simulink model "q_heli3d_semestral_project_FL"  (Simulink 8.9)
settings: Solver=ode1  StartTime=0.0  StopTime=inf  FixedStep=0.002  RelTol=1e-3  EnableMultiTasking=on
values from neighbouring files (symbols this model uses):
  ae1 = model_identified.Parameters(3).Value    [model_benchmark_init.m]    (also in workspace.mat = 1.36231449822)
  ae2 = model_identified.Parameters(4).Value    [model_benchmark_init.m]    (also in workspace.mat = -0.378717172069)
  at = model_identified.Parameters(7).Value    [model_benchmark_init.m]    (also in workspace.mat = -0.463804529993)
  be = model_identified.Parameters(6).Value    [model_benchmark_init.m]    (also in workspace.mat = 0.116311837295)
  bl = model_identified.Parameters(2).Value    [model_benchmark_init.m]    (also in workspace.mat = 0.103160863637)
  bt = model_identified.Parameters(9).Value    [model_benchmark_init.m]    (also in workspace.mat = 0.962119048974)
  ce = model_identified.Parameters(5).Value    [model_benchmark_init.m]    (also in workspace.mat = 0.04469700002)
  cl = model_identified.Parameters(1).Value    [model_benchmark_init.m]    (also in workspace.mat = 0.202457747385)
  ct = model_identified.Parameters(8).Value    [model_benchmark_init.m]    (also in workspace.mat = 0.00762763482449)
  elev_0 = -0.479965544298    [workspace.mat]
  K_AMP = 3    [workspace.mat]
  K_EC_E = -0.00153398078789    [workspace.mat]
  K_EC_P = 0.00153398078789    [workspace.mat]
  K_EC_T = 0.000766990393943    [workspace.mat]
  par_ctrl =     [workspace.mat]
  par_id = struct    [model_benchmark_init.m]    (also in workspace.mat = )
  VMAX_AMP = 24    [workspace.mat]
  VMAX_DAC = 10    [workspace.mat]
  wcf = 125.663706144    [workspace.mat]
  x0 = [0; 0; 0; 0; 0; 0]    [model_benchmark_init.m]    (also in model_benchmark_ode45.m = [0; 0; 0; 0; 0.1; 0]; workspace.mat = [0 0 0.1745 0 -0.1047 0])
  zetaf = 0.9    [workspace.mat]
undefined symbols (not defined in the file or in its folder): HIL, qc_get_step_size
libraries: quarc_library x4, simulink_extras x4
settings Model: Creator=MLevis  LastModifiedBy=obrusvit  SimulationMode=external  ExtModeTrigDuration=1000000
settings SolverCC: PositivePriorityOrder=on
settings DataIOCC: MaxDataPoints=100000
settings OptimizationCC: ExpressionDepthLimit=2147483647  InitFltsAndDblsToZero=on
settings DebuggingCC: SaveWithParameterizedLinksMsg=none  SolverPrmCheckMsg=warning
settings RTWCC: SystemTargetFile=quarc_win64.tlc  TemplateMakefile=quarc_default_tmf  Description=QUARC Win64 Target
settings STFCustomTargetCC: TargetPreCompLibLocation=C:\PROGRA~3\QUARC\lib\2017a\win64\release  ConcurrentExecutionCompliant=on  GeneratePreprocessorConditionals=Disable all  SystemTargetFile=quarc_win64.tlc
settings GRTTargetCC: TargetPreCompLibLocation=C:\PROGRA~3\QUARC\lib\2017a\win64\release  ParMdlRefBuildCompliant=off  CompOptLevelCompliant=off  MatFileLogging=off  CPPClassGenCompliant=off  UseToolchainInfoCompliant=off  ExtMode=on  ExtModeMexFile=quarc_comm

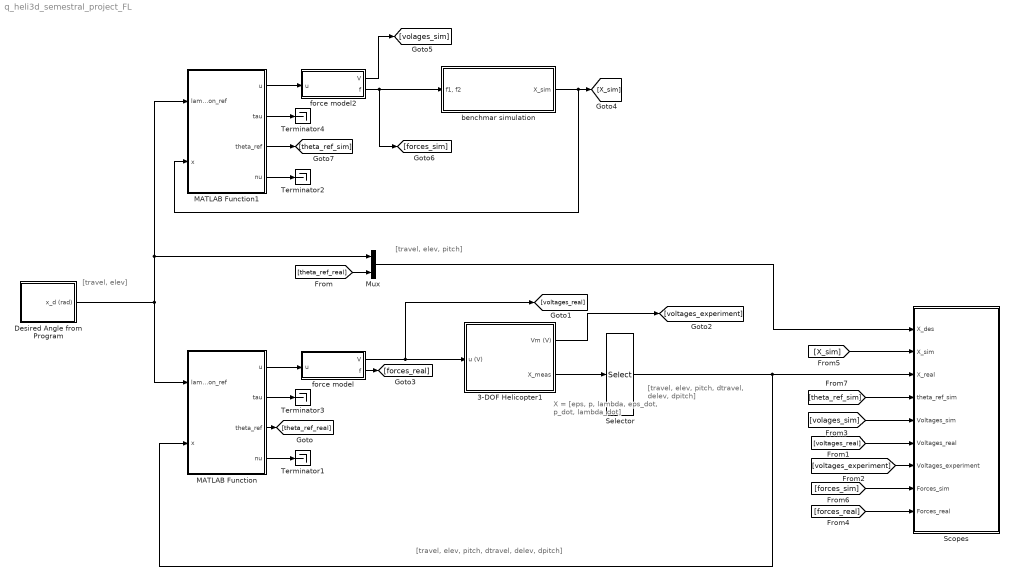
== system q_heli3d_semestral_project_FL ==
  note: [travel, elev]
  note: [travel, elev, pitch, dtravel, delev, dpitch]
  note: [travel, elev, pitch]
  note: X = [eps, p, lambda, eps_dot, p_dot, lambda_dot]
  note: [travel, elev, pitch, dtravel, delev, dpitch]
  3-DOF Helicopter1 : Subsystem
  Desired Angle from Program : Subsystem
  MATLAB Function : MATLAB Function  TreatAsAtomicUnit=on
  MATLAB Function1 : MATLAB Function  TreatAsAtomicUnit=on
  Mux : Mux  Inputs=2
  Scopes : Subsystem
  Selector : Selector  InputPortWidth=6  IndexOptions=Index vector (dialog)  Indices=[3 1 2 6 4 5]  OutputSizes=1
  Terminator{1..4} (4 alike) : Terminator
  benchmar simulation : Subsystem
  force model : Subsystem
  force model2 : Subsystem
  wires:
  Mux/1 -> Scopes/1(X_des)
  [theta_ref_real] -> Mux/2
  MATLAB Function/2(tau) -> Terminator3/1
  MATLAB Function/4(nu) -> Terminator1/1
  force model/2(f) -> [forces_real]
  MATLAB Function/3(theta_ref) -> [theta_ref_real]
  Desired Angle from Program/1(x_d (rad)) -> MATLAB Function/1(lambda_epsilon_ref), Mux/1, MATLAB Function1/1(lambda_epsilon_ref)
  [forces_real] -> Scopes/9("Forces_real ")
  [voltages_real] -> Scopes/6("Voltages_real ")
  MATLAB Function/1(u) -> force model/1(u)
  3-DOF Helicopter1/2(X_meas) -> Selector/1
  Selector/1 -> MATLAB Function/2(x), Scopes/3("X_real ")
  [X_sim] -> Scopes/2(X_sim)
  force model2/2(f) -> benchmar simulation/1("f1, f2"), [forces_sim]
  benchmar simulation/1("X_sim ") -> MATLAB Function1/2(x), [X_sim]
  force model/1(V) -> [voltages_real], 3-DOF Helicopter1/1(u (V))
  MATLAB Function1/1(u) -> force model2/1(u)
  MATLAB Function1/4(nu) -> Terminator2/1
  MATLAB Function1/3(theta_ref) -> [theta_ref_sim]
  MATLAB Function1/2(tau) -> Terminator4/1
  force model2/1(V) -> [volages_sim]
  [volages_sim] -> Scopes/5(Voltages_sim)
  [forces_sim] -> Scopes/8(Forces_sim)
  [theta_ref_sim] -> Scopes/4("theta_ref_sim ")
  3-DOF Helicopter1/1(Vm (V)) -> [voltages_experiment]
  [voltages_experiment] -> Scopes/7(Voltages_experiment)

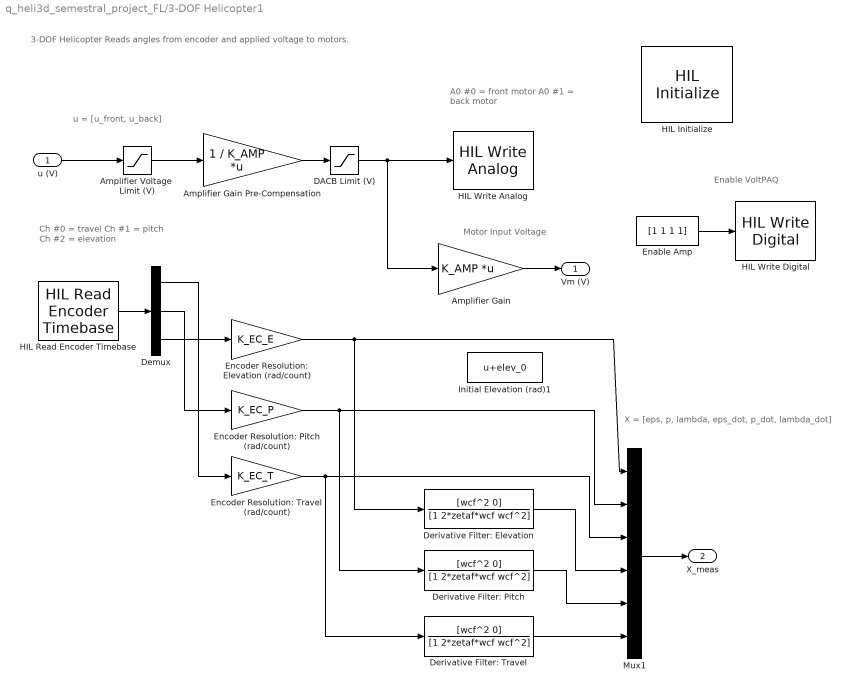
== system q_heli3d_semestral_project_FL/3-DOF Helicopter1 ==
  note: Enable VoltPAQ
  note: X = [eps, p, lambda, eps_dot, p_dot, lambda_dot]
  note: Ch #0 = travel
      | Ch #1 = pitch
      | Ch #2 = elevation
  note: 3-DOF Helicopter
      | Reads angles from encoder and applied voltage to motors.
  note: Motor Input Voltage
  note: u = [u_front, u_back]
  note: A0 #0 = front motor
      | A0 #1 = back motor
  u (V) : Inport
  Amplifier Gain : Gain  Gain=K_AMP  Multiplication=Matrix(K*u)  SaturateOnIntegerOverflow=on  OutDataTypeStr=Inherit: Same as input  ParamDataTypeStr=Inherit: Same as input
  Amplifier Gain Pre-Compensation : Gain  Gain=1 / K_AMP  Multiplication=Matrix(K*u)  SaturateOnIntegerOverflow=on  OutDataTypeStr=Inherit: Same as input  ParamDataTypeStr=Inherit: Same as input
  Amplifier Voltage  Limit (V) : Saturate  UpperLimit=VMAX_AMP  LowerLimit=-VMAX_AMP
  DACB Limit (V) : Saturate  UpperLimit=VMAX_DAC  LowerLimit=-VMAX_DAC
  Demux : Demux  Outputs=3
  Derivative Filter: Elevation : TransferFcn  Numerator=[wcf^2 0]  Denominator=[1 2*zetaf*wcf wcf^2]
  Derivative Filter: Pitch : TransferFcn  Numerator=[wcf^2 0]  Denominator=[1 2*zetaf*wcf wcf^2]
  Derivative Filter: Travel : TransferFcn  Numerator=[wcf^2 0]  Denominator=[1 2*zetaf*wcf wcf^2]
  Enable Amp : Constant  Value=[1 1 1 1]
  Encoder Resolution: Elevation (rad/count) : Gain  Gain=K_EC_E
  Encoder Resolution: Pitch (rad/count) : Gain  Gain=K_EC_P
  Encoder Resolution: Travel (rad/count) : Gain  Gain=K_EC_T
  HIL Initialize : quarc_library/Data Acquisition/Generic/Configuration/HIL Initialize  object_name=HIL-1  board_type=q8_usb  board_number=0  board_options=update_rate=normal;decimation=1  exclusive=off  active=on  hardware_clocks=[0:2]  clock_modes=[]  initial_clock_frequencies=[]  set_clock_params_at_start=off  set_clock_params_at_switch_in=off  set_clock_frequencies_at_start=off  set_clock_frequencies_at_switch_in=off  analog_input_channels=[0:7]  analog_input_configurations=[]  analog_input_maximums=10  analog_input_minimums=-10  set_analog_input_params_at_start=on  set_analog_input_params_at_switch_in=off  analog_output_channels=[0:7]  analog_output_maximums=10  analog_output_minimums=-10  initial_analog_outputs=[0]  final_analog_outputs=[0]  watchdog_analog_outputs=0  set_analog_output_params_at_start=on  set_analog_output_params_at_switch_in=off  set_analog_outputs_at_start=on  set_analog_outputs_at_switch_in=off  set_analog_outputs_at_terminate=on  set_analog_outputs_at_switch_out=off  set_analog_outputs_on_watchdog=off  digital_input_channels=[]  digital_output_channels=[]  digital_output_configuration=[]  initial_digital_outputs=[1]  final_digital_outputs=[1]  watchdog_digital_outputs=[1]  set_digital_output_params_at_start=off  set_digital_output_params_at_switch_in=off  set_digital_outputs_at_start=on  set_digital_outputs_at_switch_in=off  set_digital_outputs_at_terminate=on  set_digital_outputs_at_switch_out=off  set_digital_outputs_on_watchdog=off  encoder_channels=[0:7]  quadrature=[4]  encoder_filter_frequency=[]  initial_encoder_counts=[0]  set_encoder_params_at_start=on  set_encoder_params_at_switch_in=off  set_encoder_counts_at_start=on  set_encoder_counts_at_switch_in=off  pwm_channels=[0:7]  pwm_modes=0  pwm_frequency=99.532799999999995e6/4095  pwm_configuration=[0]  pwm_alignment=[0]  pwm_polarity=[1]  pwm_leading_deadband=[0]  pwm_trailing_deadband=[0]  initial_pwm_outputs=[0]  final_pwm_outputs=[0]  watchdog_pwm_outputs=[0]  set_pwm_params_at_start=on  set_pwm_params_at_switch_in=off  set_pwm_outputs_at_start=on  set_pwm_outputs_at_switch_in=off  set_pwm_outputs_at_terminate=on  set_pwm_outputs_at_switch_out=off  set_pwm_outputs_on_watchdog=off  other_output_channels=[]  initial_other_outputs=[]  final_other_outputs=[]  watchdog_other_outputs=[]  set_other_outputs_at_start=off  set_other_outputs_at_switch_in=off  set_other_outputs_at_terminate=off  set_other_outputs_at_switch_out=off  set_other_outputs_on_watchdog=off
  HIL Read Encoder Timebase : quarc_library/Data Acquisition/Generic/Timebases/HIL Read Encoder Timebase  object_name=HIL-1  clock=0  channels=[0:2]  samples_in_buffer=max(ceil(1/qc_get_step_size), 1)  active=on  vector_output=on  data_type_mode=Inherit via back propagation  data_type=double
  HIL Write Analog : quarc_library/Data Acquisition/Generic/Immediate I//O/HIL Write Analog  object_name=HIL-1  channels=[0,1]  sample_time=-1  active=off  vector_input=on
  HIL Write Digital : quarc_library/Data Acquisition/Generic/Immediate I//O/HIL Write Digital  object_name=HIL-1  channels=[0:3]  sample_time=-1  active=off  vector_input=on
      settings: SourceProductName=QUARC Targets
  Initial Elevation (rad)1 : Bias  Bias=elev_0
  Mux1 : Mux  Inputs=6
  Vm (V) : Outport
  X_meas : Outport  Port=2
  wires:
  Enable Amp/1 -> HIL Write Digital/1
  Encoder Resolution: Elevation (rad/count)/1 -> Mux1/1, Derivative Filter: Elevation/1
  Derivative Filter: Travel/1 -> Mux1/6
  Derivative Filter: Pitch/1 -> Mux1/5
  Derivative Filter: Elevation/1 -> Mux1/4
  Encoder Resolution: Travel (rad/count)/1 -> Derivative Filter: Travel/1, Mux1/3
  Encoder Resolution: Pitch (rad/count)/1 -> Derivative Filter: Pitch/1, Mux1/2
  Demux/2 -> Encoder Resolution: Pitch (rad/count)/1
  Demux/1 -> Encoder Resolution: Travel (rad/count)/1
  Demux/3 -> Encoder Resolution: Elevation (rad/count)/1
  DACB Limit (V)/1 -> HIL Write Analog/1, Amplifier Gain/1
  u (V)/1 -> Amplifier Voltage  Limit (V)/1
  Amplifier Gain/1 -> Vm (V)/1
  Amplifier Voltage  Limit (V)/1 -> Amplifier Gain Pre-Compensation/1
  Amplifier Gain Pre-Compensation/1 -> DACB Limit (V)/1
  Mux1/1 -> X_meas/1
  HIL Read Encoder Timebase/1 -> Demux/1

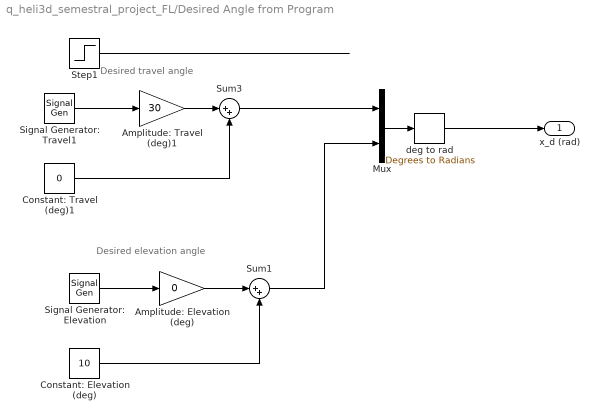
== system q_heli3d_semestral_project_FL/Desired Angle from Program ==
  note: Desired elevation angle
  note: Desired travel angle
  Amplitude: Elevation (deg) : Gain  Gain=0
  Amplitude: Travel (deg)1 : Gain  Gain=30
  Constant: Elevation (deg) : Constant  Value=10
  Constant: Travel (deg)1 : Constant  Value=0
  Mux : Mux  Inputs=2
  Signal Generator: Elevation : SignalGenerator  WaveForm=square  Frequency=0.04
  Signal Generator: Travel1 : SignalGenerator  WaveForm=square  Frequency=0.02
  Step1 : Step  Time=20  After=180  SampleTime=0
  Sum1 : Sum  Inputs=|++
  Sum3 : Sum  Inputs=|++
  deg to rad : simulink_extras/Transformations/Degrees to Radians
  x_d (rad) : Outport
  wires:
  Mux/1 -> deg to rad/1
  Constant: Elevation (deg)/1 -> Sum1/2
  Amplitude: Elevation (deg)/1 -> Sum1/1
  Signal Generator: Elevation/1 -> Amplitude: Elevation (deg)/1
  Sum1/1 -> Mux/2
  deg to rad/1 -> x_d (rad)/1
  Sum3/1 -> Mux/1
  Signal Generator: Travel1/1 -> Amplitude: Travel (deg)1/1
  Constant: Travel (deg)1/1 -> Sum3/2
  Amplitude: Travel (deg)1/1 -> Sum3/1
  Step1/1 -> ?

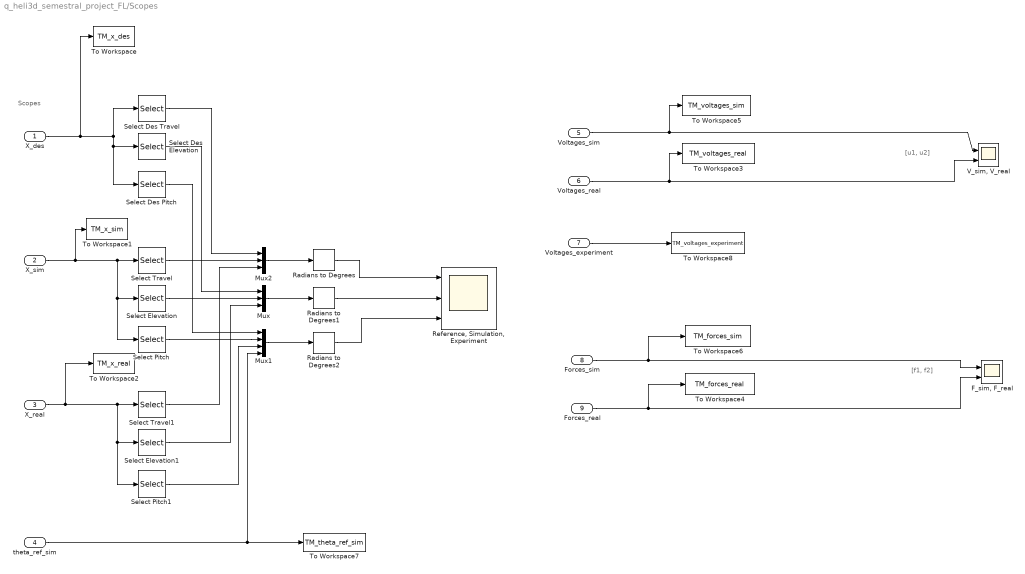
== system q_heli3d_semestral_project_FL/Scopes ==
  note: Scopes
  note: [f1, f2]
  note: [u1, u2]
  X_des : Inport
  X_sim : Inport  Port=2
  "X_real " : Inport  Port=3
  "theta_ref_sim " : Inport  Port=4
  Voltages_sim : Inport  Port=5
  "Voltages_real " : Inport  Port=6
  Voltages_experiment : Inport  Port=7
  Forces_sim : Inport  Port=8
  "Forces_real " : Inport  Port=9
  "F_sim, F_real" : Scope  NumInputPorts=2
  Mux : Mux  Inputs=3
  Mux1 : Mux
  Mux2 : Mux  Inputs=3
  Radians to Degrees : simulink_extras/Transformations/Radians to Degrees
  Radians to Degrees1 : simulink_extras/Transformations/Radians to Degrees
  Radians to Degrees2 : simulink_extras/Transformations/Radians to Degrees
  "Reference, Simulation, Experiment" : Scope  NumInputPorts=3
  Select Des Elevation : Selector  InputPortWidth=3  IndexOptions=Index vector (dialog)  Indices=2  OutputSizes=1
  Select Des Pitch : Selector  InputPortWidth=3  IndexOptions=Index vector (dialog)  Indices=3  OutputSizes=1
  Select Des Travel : Selector  InputPortWidth=3  IndexOptions=Index vector (dialog)  Indices=1  OutputSizes=1
  Select Elevation : Selector  InputPortWidth=6  IndexOptions=Index vector (dialog)  Indices=2  OutputSizes=1
  Select Elevation1 : Selector  InputPortWidth=6  IndexOptions=Index vector (dialog)  Indices=2  OutputSizes=1
  Select Pitch : Selector  InputPortWidth=6  IndexOptions=Index vector (dialog)  Indices=3  OutputSizes=1
  Select Pitch1 : Selector  InputPortWidth=6  IndexOptions=Index vector (dialog)  Indices=3  OutputSizes=1
  Select Travel : Selector  InputPortWidth=6  IndexOptions=Index vector (dialog)  Indices=1  OutputSizes=1
  Select Travel1 : Selector  InputPortWidth=6  IndexOptions=Index vector (dialog)  Indices=1  OutputSizes=1
  To Workspace : ToWorkspace  VariableName=TM_x_des  SampleTime=-1
  To Workspace1 : ToWorkspace  VariableName=TM_x_sim  SampleTime=-1
  To Workspace2 : ToWorkspace  VariableName=TM_x_real  SampleTime=-1
  To Workspace3 : ToWorkspace  VariableName=TM_voltages_real  SampleTime=-1
  To Workspace4 : ToWorkspace  VariableName=TM_forces_real  SampleTime=-1
  To Workspace5 : ToWorkspace  VariableName=TM_voltages_sim  SampleTime=-1
  To Workspace6 : ToWorkspace  VariableName=TM_forces_sim  SampleTime=-1
  To Workspace7 : ToWorkspace  VariableName=TM_theta_ref_sim  SampleTime=-1
  To Workspace8 : ToWorkspace  VariableName=TM_voltages_experiment  SampleTime=-1
  "V_sim, V_real" : Scope  NumInputPorts=2
  wires:
  Mux1/1 -> Radians to Degrees2/1
  X_sim/1 -> To Workspace1/1, Select Pitch/1, Select Elevation/1, Select Travel/1
  Mux2/1 -> Radians to Degrees/1
  Select Elevation/1 -> Mux/2
  Select Pitch/1 -> Mux1/2
  Select Travel/1 -> Mux2/2
  X_des/1 -> To Workspace/1, Select Des Pitch/1, Select Des Elevation/1, Select Des Travel/1
  Select Des Elevation/1 -> Mux/1
  Select Des Travel/1 -> Mux2/1
  Select Des Pitch/1 -> Mux1/1
  Mux/1 -> Radians to Degrees1/1
  "Voltages_real "/1 -> To Workspace3/1, "V_sim, V_real"/2
  "Forces_real "/1 -> To Workspace4/1, "F_sim, F_real"/2
  "X_real "/1 -> To Workspace2/1, Select Pitch1/1, Select Elevation1/1, Select Travel1/1
  Select Travel1/1 -> Mux2/3
  Select Elevation1/1 -> Mux/3
  Select Pitch1/1 -> Mux1/3
  Radians to Degrees/1 -> "Reference, Simulation, Experiment"/1
  Radians to Degrees1/1 -> "Reference, Simulation, Experiment"/2
  Radians to Degrees2/1 -> "Reference, Simulation, Experiment"/3
  Voltages_sim/1 -> To Workspace5/1, "V_sim, V_real"/1
  Forces_sim/1 -> To Workspace6/1, "F_sim, F_real"/1
  "theta_ref_sim "/1 -> To Workspace7/1, Mux1/4
  Voltages_experiment/1 -> To Workspace8/1

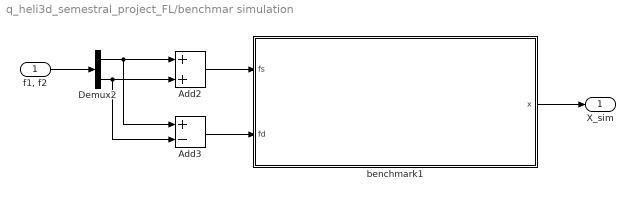
== system q_heli3d_semestral_project_FL/benchmar simulation ==
  "f1, f2" : Inport
  Add2 : Sum
  Add3 : Sum  Inputs=+-
  Demux2 : Demux  Outputs=2
  benchmark1 : Subsystem
  "X_sim " : Outport
  wires:
  Add3/1 -> benchmark1/2("fd ")
  Demux2/1 -> Add3/1, Add2/1
  Add2/1 -> benchmark1/1("fs ")
  Demux2/2 -> Add3/2, Add2/2
  "f1, f2"/1 -> Demux2/1
  benchmark1/1(x) -> "X_sim "/1

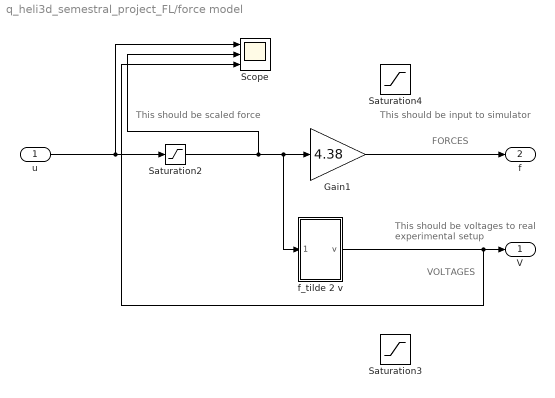
== system q_heli3d_semestral_project_FL/force model ==
  note: This should be voltages to
      |  real experimental setup
  note: This should be scaled force
  note: This should be input to simulator
  note: FORCES
  note: VOLTAGES
  u : Inport
  Gain1 : Gain  Gain=4.38
  Saturation2 : Saturate  UpperLimit=1  LowerLimit=-0.23
  Saturation3 : Saturate  UpperLimit=24  LowerLimit=0
  Saturation4 : Saturate  UpperLimit=inf  LowerLimit=0
  Scope : Scope  NumInputPorts=3
  f_tilde 2 v : Subsystem
  V : Outport
  f : Outport  Port=2
  wires:
  u/1 -> Saturation2/1, Scope/1
  Saturation2/1 -> Scope/2, Gain1/1, f_tilde 2 v/1(f_tilde)
  Gain1/1 -> f/1
  f_tilde 2 v/1(v) -> Scope/3, V/1

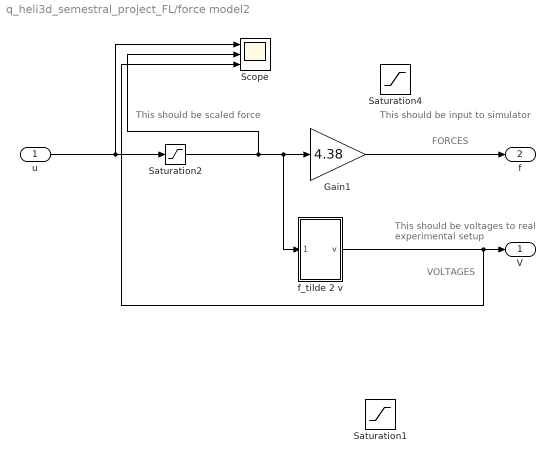
== system q_heli3d_semestral_project_FL/force model2 ==
  note: This should be voltages to
      |  real experimental setup
  note: This should be scaled force
  note: This should be input to simulator
  note: FORCES
  note: VOLTAGES
  u : Inport
  Gain1 : Gain  Gain=4.38
  Saturation1 : Saturate  UpperLimit=24  LowerLimit=0
  Saturation2 : Saturate  UpperLimit=1  LowerLimit=-0.23
  Saturation4 : Saturate  UpperLimit=inf  LowerLimit=0
  Scope : Scope  NumInputPorts=3
  f_tilde 2 v : Subsystem
  V : Outport
  f : Outport  Port=2
  wires:
  u/1 -> Saturation2/1, Scope/1
  Saturation2/1 -> Scope/2, Gain1/1, f_tilde 2 v/1(f_tilde)
  Gain1/1 -> f/1
  f_tilde 2 v/1(v) -> Scope/3, V/1

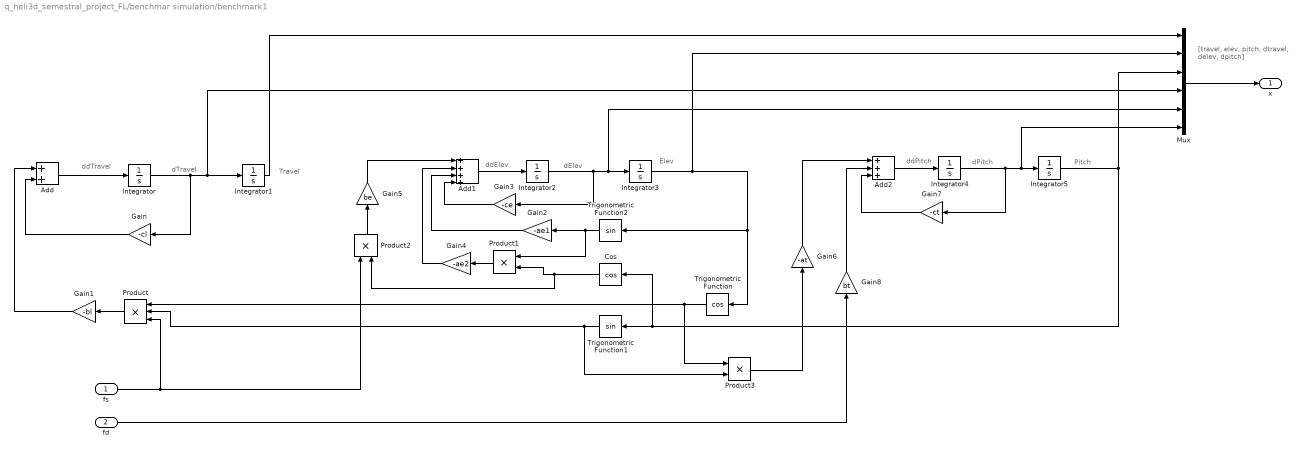
== system q_heli3d_semestral_project_FL/benchmar simulation/benchmark1 ==
  note: Pitch
  note: dPitch
  note: ddPitch
  note: Elev
  note: dElev
  note: ddElev
  note: Travel
  note: dTravel
  note: ddTravel
  note: [travel, elev, pitch, dtravel, delev, dpitch]
  "fs " : Inport
  "fd " : Inport  Port=2
  Add : Sum
  Add1 : Sum  Inputs=++++
  Add2 : Sum  Inputs=+++
  Cos : Trigonometry  Operator=cos
  Gain : Gain  Gain=-cl
  Gain1 : Gain  Gain=-bl
  Gain2 : Gain  Gain=-ae1
  Gain3 : Gain  Gain=-ce
  Gain4 : Gain  Gain=-ae2
  Gain5 : Gain  Gain=be
  Gain6 : Gain  Gain=-at
  Gain7 : Gain  Gain=-ct
  Gain8 : Gain  Gain=bt
  Integrator : Integrator  InitialCondition=x0(2)
  Integrator1 : Integrator  InitialCondition=x0(1)
  Integrator2 : Integrator  InitialCondition=x0(4)
  Integrator3 : Integrator  InitialCondition=x0(3)
  Integrator4 : Integrator  InitialCondition=x0(6)
  Integrator5 : Integrator  InitialCondition=x0(5)
  Mux : Mux  Inputs=6
  Product : Product  Inputs=3
  Product1 : Product
  Product2 : Product
  Product3 : Product
  Trigonometric Function : Trigonometry  Operator=cos
  Trigonometric Function1 : Trigonometry
  Trigonometric Function2 : Trigonometry
  x : Outport
  wires:
  Gain5/1 -> Add1/1
  Product/1 -> Gain1/1
  Product2/1 -> Gain5/1
  "fd "/1 -> Gain8/1
  Trigonometric Function/1 -> Product3/1, Product/1
  Product3/1 -> Gain6/1
  Gain7/1 -> Add2/3
  Cos/1 -> Product2/2, Product1/2
  Gain4/1 -> Add1/2
  Gain2/1 -> Add1/3
  Mux/1 -> x/1
  Gain8/1 -> Add2/2
  Add2/1 -> Integrator4/1
  Gain6/1 -> Add2/1
  Integrator1/1 -> Mux/1
  Gain1/1 -> Add/1
  Integrator3/1 -> Mux/2, Trigonometric Function2/1, Trigonometric Function/1
  Integrator2/1 -> Gain3/1, Mux/5, Integrator3/1
  Product1/1 -> Gain4/1
  Gain3/1 -> Add1/4
  Integrator4/1 -> Gain7/1, Mux/6, Integrator5/1
  Integrator/1 -> Gain/1, Mux/4, Integrator1/1
  Gain/1 -> Add/2
  Add1/1 -> Integrator2/1
  Integrator5/1 -> Mux/3, Cos/1, Trigonometric Function1/1
  Trigonometric Function2/1 -> Product1/1, Gain2/1
  Trigonometric Function1/1 -> Product3/2, Product/2
  "fs "/1 -> Product2/1, Product/3
  Add/1 -> Integrator/1

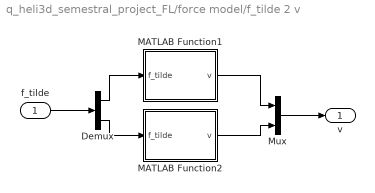
== system q_heli3d_semestral_project_FL/force model/f_tilde 2 v ==
  f_tilde : Inport
  Demux : Demux  Outputs=2
  MATLAB Function1 : MATLAB Function  TreatAsAtomicUnit=on
  MATLAB Function2 : MATLAB Function  TreatAsAtomicUnit=on
  Mux : Mux  Inputs=2
  v : Outport
  wires:
  f_tilde/1 -> Demux/1
  Mux/1 -> v/1
  Demux/1 -> MATLAB Function1/1(f_tilde)
  Demux/2 -> MATLAB Function2/1(f_tilde)
  MATLAB Function1/1(v) -> Mux/1
  MATLAB Function2/1(v) -> Mux/2

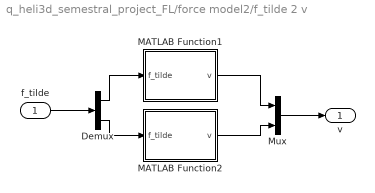
== system q_heli3d_semestral_project_FL/force model2/f_tilde 2 v ==
  f_tilde : Inport
  Demux : Demux  Outputs=2
  MATLAB Function1 : MATLAB Function  TreatAsAtomicUnit=on
  MATLAB Function2 : MATLAB Function  TreatAsAtomicUnit=on
  Mux : Mux  Inputs=2
  v : Outport
  wires:
  f_tilde/1 -> Demux/1
  Mux/1 -> v/1
  Demux/1 -> MATLAB Function1/1(f_tilde)
  Demux/2 -> MATLAB Function2/1(f_tilde)
  MATLAB Function1/1(v) -> Mux/1
  MATLAB Function2/1(v) -> Mux/2

== matlab function force model/f_tilde 2 v/MATLAB Function2 ==
  data: f_tilde input double; v output double; par_inputs parameter double
function v = fcn(f_tilde, par_inputs)

v = scaled_force_2_voltage(f_tilde, par_inputs.scaled_f_2_v_par, par_inputs.scaled_f_2_v_ths);

== matlab function MATLAB Function ==
  data: lambda_epsilon_ref input double; x input double; u output double; tau output double; theta_ref output double; nu output double; par_id parameter double; par_ctrl parameter double
function [u, tau, theta_ref, nu] = fcn(lambda_epsilon_ref, x, par_id, par_ctrl)

T = diag([-par_id.bl*cos(x(2)), par_id.be, par_id.bt]);

g_bar = [0;...
         sin(x(2))*(par_id.ae1+par_id.ae2*cos(x(3)))*0.95;...
         par_id.at*cos(x(2))*sin(x(3))];

R_bar = diag([par_id.cl, par_id.ce, par_id.ct]);
                    

nu = [0;0;0];

nu(1:2) = pinv(T(1:2, 1:2)) * ( g_bar(1:2)   -   par_ctrl.Omega(1:2,1:2)^2 * (x(1:2)-lambda_epsilon_ref)   +   (R_bar(1:2,1:2) - par_ctrl.Xi(1:2,1:2)) * x(4:5) );
% nu(1) = nu(1) - 0.12;
nu(1) = nu(1);


theta_ref = atan2( nu(1), nu(2) );

if abs(x(2)<deg2rad(1))
    theta_ref = 0;
end


nu(3)   = pinv(T(3, 3)) * (g_bar(3)   -   par_ctrl.Omega(3,3)^2 * (x(3)-theta_ref)   +   (R_bar(3,3) - par_ctrl.Xi(3,3)) * x(6));

B = [sin(x(3)) 0;...
      cos(x(3)) 0;...
     0          1];
tau = B'*nu;

u = [1/2  1/2;...
     1/2 -1/2]* tau;

== matlab function force model/f_tilde 2 v/MATLAB Function1 ==
  data: f_tilde input double; v output double; par_inputs parameter double
function v = fcn(f_tilde, par_inputs)

v = scaled_force_2_voltage(f_tilde, par_inputs.scaled_f_2_v_par, par_inputs.scaled_f_2_v_ths);

== matlab function MATLAB Function1 ==
  data: lambda_epsilon_ref input double; x input double; u output double; tau output double; theta_ref output double; nu output double; par_id parameter double; par_ctrl parameter double
function [u, tau, theta_ref, nu] = fcn(lambda_epsilon_ref, x, par_id, par_ctrl)

T = diag([-par_id.bl*cos(x(2)), par_id.be, par_id.bt]);

g_bar = [0;...
         sin(x(2))*(par_id.ae1+par_id.ae2*cos(x(3)))*0.95;...
         par_id.at*cos(x(2))*sin(x(3))];

R_bar = diag([par_id.cl, par_id.ce, par_id.ct]);
                    

nu = [0;0;0];

nu(1:2) = pinv(T(1:2, 1:2)) * ( g_bar(1:2)   -   par_ctrl.Omega(1:2,1:2)^2 * (x(1:2)-lambda_epsilon_ref)   +   (R_bar(1:2,1:2) - par_ctrl.Xi(1:2,1:2)) * x(4:5) );
% nu(1) = nu(1) - 0.12;
nu(1) = nu(1);


theta_ref = atan2( nu(1), nu(2) );

if abs(x(2)<deg2rad(1))
    theta_ref = 0;
end


nu(3)   = pinv(T(3, 3)) * (g_bar(3)   -   par_ctrl.Omega(3,3)^2 * (x(3)-theta_ref)   +   (R_bar(3,3) - par_ctrl.Xi(3,3)) * x(6));

B = [sin(x(3)) 0;...
      cos(x(3)) 0;...
     0          1];
tau = B'*nu;

u = [1/2  1/2;...
     1/2 -1/2]* tau;

== matlab function force model2/f_tilde 2 v/MATLAB Function1 ==
  data: f_tilde input double; v output double; par_inputs parameter double
function v = fcn(f_tilde, par_inputs)

v = scaled_force_2_voltage(f_tilde, par_inputs.scaled_f_2_v_par, par_inputs.scaled_f_2_v_ths);

== matlab function force model2/f_tilde 2 v/MATLAB Function2 ==
  data: f_tilde input double; v output double; par_inputs parameter double
function v = fcn(f_tilde, par_inputs)

v = scaled_force_2_voltage(f_tilde, par_inputs.scaled_f_2_v_par, par_inputs.scaled_f_2_v_ths);
